simulink model "Rifai"  (R2017b)
settings: Solver=ode113  StartTime=0.0  StopTime=100  FixedStep=2.0  MaxStep=2.0  RelTol=1e-3
settings Model: Creator=Jimmy  LastModifiedBy=Jimmy

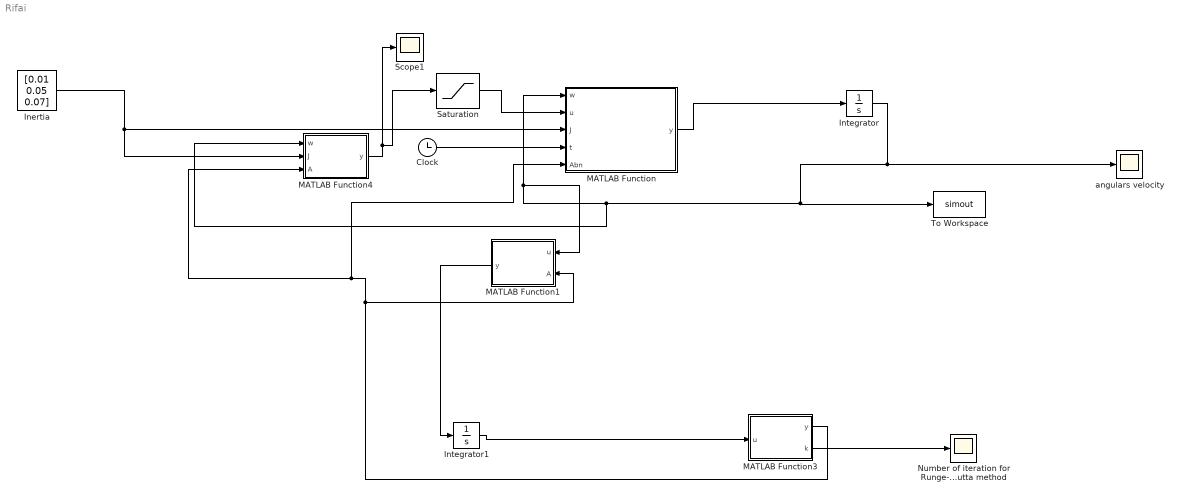
== system Rifai ==
  Clock : Clock
  "Inertia " : Constant  Tag=J  Description=J  Value=[0.01 0.05 0.07]
  Integrator : Integrator  InitialCondition=[0.03 0.01 0.02]
  Integrator1 : Integrator  InitialCondition=[-0.782 0 -0.6233; 0.6233 0 -0.782; 0 -1 0]
  MATLAB Function : MATLAB Function  TreatAsAtomicUnit=on
  MATLAB Function1 : MATLAB Function  TreatAsAtomicUnit=on
  MATLAB Function3 : MATLAB Function  TreatAsAtomicUnit=on
  MATLAB Function4 : MATLAB Function  TreatAsAtomicUnit=on
  Number of iteration for Runge-Kutta method : Scope
  Saturation : Saturate  UpperLimit=0.1  LowerLimit=-0.1  LinearizeAsGain=off  ZeroCross=off
  Scope1 : Scope
  To Workspace : ToWorkspace  VariableName=simout  SampleTime=-1
  "angulars velocity " : Scope
  wires:
  MATLAB Function3/1(y) -> MATLAB Function/5(Abn), MATLAB Function4/3(A), MATLAB Function1/2(A)
  Integrator/1 -> To Workspace/1, MATLAB Function4/1(w), MATLAB Function/1(w), MATLAB Function1/1(u), "angulars velocity "/1
  Integrator1/1 -> MATLAB Function3/1(u)
  MATLAB Function/1(y) -> Integrator/1
  MATLAB Function1/1(y) -> Integrator1/1
  "Inertia "/1 -> MATLAB Function/3(J), MATLAB Function4/2(J)
  MATLAB Function4/1(y) -> Saturation/1, Scope1/1
  MATLAB Function3/2(k) -> Number of iteration for Runge-Kutta method/1
  Clock/1 -> MATLAB Function/4(t)
  Saturation/1 -> MATLAB Function/2(u)

== matlab function Rifai/MATLAB Function1 ==
  data: u input; y output; A input
function y = kinematics(u,A)


W=[0 -u(3) u(2); u(3) 0 -u(1); -u(2) -u(1) 0];

Adot=-W*A ;

y=Adot ;
end

== matlab function Rifai/MATLAB Function ==
  data: w input; u input; y output; J input; t input; Abn input
function y = euler(w,u,J,t,Abn)

%Set Data
Ix=J(1); Iy=J(2); Iz=J(3) ;
wx=w(1) ; wy=w(2); wz=w(3);
wdot=[0;0;0];
%%Gravity Gradiant
 R=42168;
 n=(398600/(R^3))^0.5 ;
Aln=[cos(n*t) sin(n*t) 0 ; -sin(n*t) cos(n*t) 0; 0 0 1];
Abl=Abn*(Aln');
c=Abl*[1;0;0];
Ma1=(3*(n^2))*((Iz-Iy)*c(3)*c(2)) ;
Ma2=(3*(n^2))*((Ix-Iz)*c(1)*c(3)) ;
Ma3=(3*(n^2))*((Iy-Ix)*c(1)*c(2));

%% Euler Equation
wdot(1)= ((Iy-Iz)/Ix)*wy*wz+u(1)/Ix+Ma1/Ix;
wdot(2)= ((Iz-Ix)/Iy)*wx*wz+u(2)/Iy+Ma2/Iy;
wdot(3)= ((Ix-Iy)/Iz)*wx*wy+u(3)/Iz+Ma3/Iz;


y = wdot;
end

== matlab function Rifai/MATLAB Function3 ==
  data: u input; y output; k output
function [y,k]  = ortho(u)

c=1; A=u; k=0;
while c>0.000001

A=(1.5.*A)-(A*(A')*A./2) ; % Runge-Kutta method
c=trace((eye(3)-(A')*A)) ; % error
k=k+1 ; %counter
end

z=k;
y=A ;

end

== matlab function Rifai/MATLAB Function4 ==
  data: w input; y output; J input; A input
function y = control(w,J,A)

% set gain
k1=0.5; k2=0.5;

% control law 
Jd=diag(J); 
K1=k1*Jd ; K2=k2*Jd;
Ad=eye(3);
Ae=A*Ad ;
Q=(Ae')-Ae ;
e=[Q(3,2) Q(1,3) Q(2,1)]';
u=-K1*w-K2*e;

y=u;
end
